simulink model "test04"  (R2021a)
settings: Solver=VariableStepAuto  StartTime=0.0  StopTime=10.0  RelTol=1e-3
libraries: spsIdealSwitchLib x6, spsSeriesRLCBranchLib x3, spsVoltageMeasurementLib x3, simulink x2, spsAsynchronousMachineSIUnitsLib x1, spsDCVoltageSourceLib x1, spsDiscreteVariableTimeDelayLib x1, spsGroundLib x1, spspowerguiLib x1
settings Model: Creator=shashank  LastModifiedBy=shashank

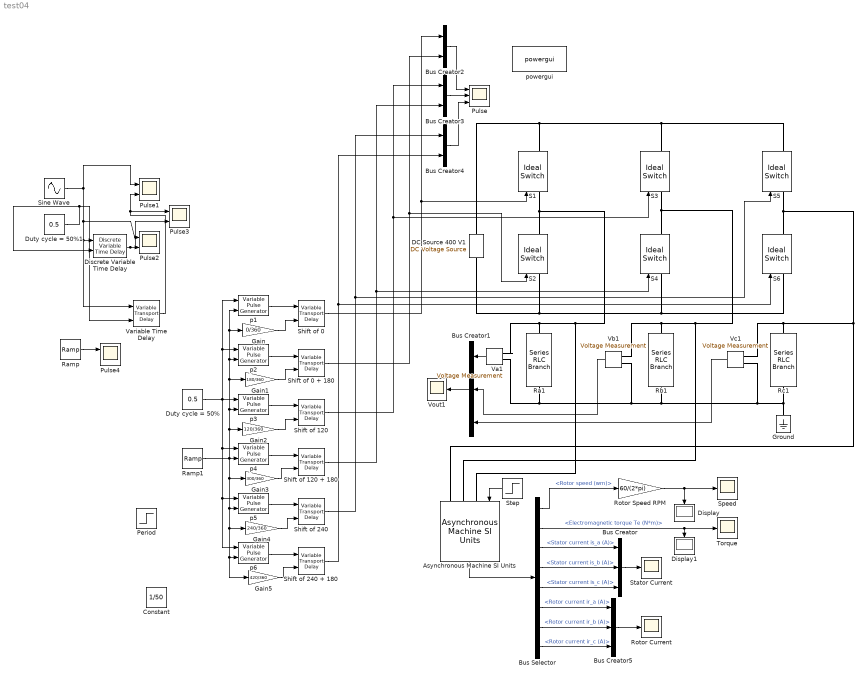
== system test04 ==
  Asynchronous Machine SI Units : spsAsynchronousMachineSIUnitsLib/Asynchronous Machine SI Units  RotorType=Squirrel-cage  PresetModel="21:  215 HP (160KW) 400 V 50Hz 1487 RPM"  MechanicalLoad=Torque Tm  ShowDetailedParameters=on  ReferenceFrame=Rotor  Units=SI  MeasurementBus=off  NominalParameters=[1.6e+05 400 50]  VoltageRatio=1  Stator=[0.01379 0.000152]  Rotor=[0.007728 0.000152]  Cage1=[0.4155 0.002066]  Cage2=[0.4168 0.0003495]  Lm=0.00769  Mechanical=[2.9 0.05658 2]  PolePairs=2  InitialConditions=[0 0 0 0 0 0 0 0]  SimulateSaturation=off  Saturation=[14.03593122, 27.81365428, 53.79336849, 72.68890987, 97.98006896, 148.6815601, 215.7428561, 302.9841135, 428.7778367 ; 230, 322, 414, 460, 506, 552, 598, 644, 690]  LoadFlowParameters=1492000  TsPowergui=0  TsBlock=-1  IterativeModel=Trapezoidal non iterative  IterativeDiscreteModel=Trapezoidal non iterative  Pmec=1.492e+006
  Bus Creator : BusCreator  Inputs=3
  Bus Creator1 : BusCreator  Inputs=3
  Bus Creator2 : BusCreator  Inputs=2
  Bus Creator3 : BusCreator  Inputs=2
  Bus Creator4 : BusCreator  Inputs=2
  Bus Creator5 : BusCreator  Inputs=3
  Bus Selector : BusSelector  OutputSignals=Mechanical.Rotor speed (wm),Mechanical.Electromagnetic torque Te (N*m),Stator measurements.Stator current is_a (A),Stator measurements.Stator current is_b (A),Stator measurements.Stator current is_c (A),Rotor measurements.Rotor current ir_a (A),Rotor measurements.Rotor current ir_b (A),Rotor measurements.Rotor current ir_c (A)
  Constant : Constant  Value=1/50
  DC Source 400 V1 : spsDCVoltageSourceLib/DC Voltage Source  Amplitude=400  Measurements=Voltage
  Discrete Variable Time Delay : spsDiscreteVariableTimeDelayLib/Discrete Variable Time Delay  MaxDelay=1  InitialValue=0  Ts=50e-6  DFT=on
      settings: SourceProductBaseCode=PS
  Display : Display
  Display1 : Display
  Duty cycle = 50% : Constant  Value=0.5
  Duty cycle = 50%1 : Constant  Value=0.5
  Gain : Gain  Gain=0/360
  Gain1 : Gain  Gain=180/360
  Gain2 : Gain  Gain=120/360
  Gain3 : Gain  Gain=300/360
  Gain4 : Gain  Gain=240/360
  Gain5 : Gain  Gain=420/360
  Ground : spsGroundLib/Ground  LConnTagsString=a
  Period : Step  Time=5  Before=1/50  After=1/25  SampleTime=0
  Pulse : Scope  NumInputPorts=3
  Pulse{1..4} (4 alike) : Scope  NumInputPorts=2
  Ra1 : spsSeriesRLCBranchLib/Series RLC Branch  LConnTagsString=__new0  RConnTagsString=__new0  BranchType=R  Resistance=10  Inductance=1e-3  SetiL0=off  InitialCurrent=0  Capacitance=1e-6  Setx0=off  InitialVoltage=0  Measurements=None
  Ramp : simulink/Sources/Ramp  slope=1/400  start=2  InitialOutput=1/50
  Ramp1 : simulink/Sources/Ramp  slope=1/400  start=2  InitialOutput=1/50
  Rb1 : spsSeriesRLCBranchLib/Series RLC Branch  LConnTagsString=__new0  RConnTagsString=__new0  BranchType=R  Resistance=10  Inductance=1e-3  SetiL0=off  InitialCurrent=0  Capacitance=1e-6  Setx0=off  InitialVoltage=0  Measurements=None
  Rc1 : spsSeriesRLCBranchLib/Series RLC Branch  LConnTagsString=__new0  RConnTagsString=__new0  BranchType=R  Resistance=10  Inductance=1e-3  SetiL0=off  InitialCurrent=0  Capacitance=1e-6  Setx0=off  InitialVoltage=0  Measurements=None
  Rotor Current : Scope
  Rotor Speed RPM : Gain  Gain=60/(2*pi)
  S{1..6} (6 alike) : spsIdealSwitchLib/Ideal Switch  Ron=1e-5  Lon=0  IC=0  Rs=1e5  Cs=inf  Measurements=on
  Shift of 0 : VariableTransportDelay  MaximumDelay=10  FixedBuffer=on  ZeroDelay=on
  Shift of 0 + 180 : VariableTransportDelay  MaximumDelay=10  FixedBuffer=on  ZeroDelay=on
  Shift of 120 : VariableTransportDelay  MaximumDelay=10  FixedBuffer=on  ZeroDelay=on
  Shift of 120 + 180 : VariableTransportDelay  MaximumDelay=10  FixedBuffer=on  ZeroDelay=on
  Shift of 240 : VariableTransportDelay  MaximumDelay=10  FixedBuffer=on  ZeroDelay=on
  Shift of 240 + 180 : VariableTransportDelay  MaximumDelay=10  FixedBuffer=on  ZeroDelay=on
  Sine Wave : Sin  SampleTime=0
  Speed : Scope
  Stator Current : Scope
  Step : Step  Time=5  Before=1000  After=1000  SampleTime=0
  Torque : Scope
  Va1 : spsVoltageMeasurementLib/Voltage Measurement  PhasorSimulation=off  OutputType=Complex  PSBequivalent=0
  Variable Time Delay : VariableTransportDelay  MaximumDelay=10  FixedBuffer=on  ZeroDelay=on
  Vb1 : spsVoltageMeasurementLib/Voltage Measurement  PhasorSimulation=off  OutputType=Complex  PSBequivalent=0
  Vc1 : spsVoltageMeasurementLib/Voltage Measurement  PhasorSimulation=off  OutputType=Complex  PSBequivalent=0
  Vout1 : Scope
  p{1..6} (6 alike) : VariablePulseGenerator  SampleTime=0.1
  powergui : spspowerguiLib/powergui  Priority=1  SimulationMode=Continuous  SampleTime=50e-6  frequency=60  Iterations=50  frequencyindice=0  Pbase=100e6  ErrMax=1e-4  UnitsV=kV  UnitsW=MW  buscounter=0  FunctionMessages=off  echomessages=off  EnableUseOfTLC=off  CurrentSourceSwitches=off  DisableSnubberDevices=off  DisableRonSwitches=off  DisableVfSwitches=off  DisplayEquations=off  AutomaticDiscreteSolvers=off  SolverType=Tustin/Backward Euler (TBE)  Interpol=off  ExternalGateDelay=off  methode=off  Ts=100  x0status=blocks  SPID=on  SwTol=0  HookPort=off  NonlinearTolerance=1e-4  nMaxIteration=100  ContinueOnMaxIteration=off  RestoreLinks=warning  ResistiveCurrentMeasurement=off  Frange=[0:2:500]  Ylog=off  Xlog=on  ShowGrid=off  save=off  variable=ZData  structure=0  ZoomFFT=off  StartTime=0.0  cycles=1  DisplayStyle=1  fundamental=60  FreqAxis=off  MaxFrequency=1000  frequencyindicesteady=1  RmsSteady=1  display=off
  wires:
  Step/1 -> Asynchronous Machine SI Units/1
  Bus Creator3/1 -> Pulse/2
  Asynchronous Machine SI Units/1 -> Bus Selector/1
  Bus Selector/7 -> Bus Creator5/2  "<Rotor current ir_b (A)>"
  Bus Selector/4 -> Bus Creator/2  "<Stator current is_b (A)>"
  Bus Creator/1 -> Stator Current/1
  Bus Creator2/1 -> Pulse/1
  Bus Selector/2 -> Torque/1, Display1/1  "<Electromagnetic torque Te (N*m)>"
  Bus Selector/6 -> Bus Creator5/1  "<Rotor current ir_a (A)>"
  Vc1/1 -> Bus Creator1/3
  Bus Selector/8 -> Bus Creator5/3  "<Rotor current ir_c (A)>"
  Va1/1 -> Bus Creator1/1
  Bus Selector/5 -> Bus Creator/3  "<Stator current is_c (A)>"
  Vb1/1 -> Bus Creator1/2
  Bus Creator1/1 -> Vout1/1
  Bus Creator5/1 -> Rotor Current/1
  Rotor Speed RPM/1 -> Speed/1, Display/1
  Bus Creator4/1 -> Pulse/3
  Bus Selector/1 -> Rotor Speed RPM/1  "<Rotor speed (wm)>"
  Bus Selector/3 -> Bus Creator/1  "<Stator current is_a (A)>"
  Ramp1/1 -> Gain2/1, Gain1/1, Gain/1, p1/2, p2/2, p3/2, Gain3/1, Gain4/1, Gain5/1, p6/2, p5/2, p4/2
  Duty cycle = 50%/1 -> p6/1, p5/1, p4/1, p1/1, p2/1, p3/1
  Sine Wave/1 -> Variable Time Delay/1, Discrete Variable Time Delay/1, Pulse2/1, Pulse1/1
  Duty cycle = 50%1/1 -> Discrete Variable Time Delay/2, Variable Time Delay/2
  Variable Time Delay/1 -> Pulse1/2, Pulse3/1
  Discrete Variable Time Delay/1 -> Pulse3/2, Pulse2/2
  p1/1 -> Shift of 0/1
  Shift of 0/1 -> S1/1, Bus Creator2/1
  p2/1 -> Shift of 0 + 180/1
  p3/1 -> Shift of 120/1
  p4/1 -> Shift of 120 + 180/1
  p5/1 -> Shift of 240/1
  p6/1 -> Shift of 240 + 180/1
  Shift of 0 + 180/1 -> S2/1, Bus Creator2/2
  Shift of 120/1 -> S3/1, Bus Creator3/1
  Shift of 120 + 180/1 -> Bus Creator3/2, S4/1
  Shift of 240/1 -> Bus Creator4/1, S5/1
  Shift of 240 + 180/1 -> Bus Creator4/2, S6/1
  Gain/1 -> Shift of 0/2
  Gain1/1 -> Shift of 0 + 180/2
  Gain2/1 -> Shift of 120/2
  Gain3/1 -> Shift of 120 + 180/2
  Gain4/1 -> Shift of 240/2
  Gain5/1 -> Shift of 240 + 180/2
  Ramp/1 -> Pulse4/1
  connections:
  Vb1/LConn1 -- Ground/LConn1 -- Rc1/LConn1 -- Vc1/LConn1 -- Rb1/LConn1 -- Ra1/LConn1 -- Va1/LConn1
  S3/LConn1 -- S4/RConn1 -- Vb1/LConn2 -- Rb1/RConn1 -- Asynchronous Machine SI Units/LConn2
  DC Source 400 V1/LConn1 -- S2/LConn1 -- S4/LConn1 -- S6/LConn1
  Va1/LConn2 -- Asynchronous Machine SI Units/LConn1 -- S1/LConn1 -- S2/RConn1 -- Ra1/RConn1
  S3/RConn1 -- S5/RConn1 -- S1/RConn1 -- DC Source 400 V1/RConn1
  Asynchronous Machine SI Units/LConn3 -- Rc1/RConn1 -- Vc1/LConn2 -- S6/RConn1 -- S5/LConn1
